simulink model "fcw_ut"  (Simulink 8.1)
settings: Solver=FixedStepDiscrete  StartTime=0.0  StopTime=10.0  FixedStep=5e-3  RelTol=1e-3
undefined symbols (not defined in the file or in its folder): VIFO_BrakePedalPressed_flg, VIFO_FCWTargetVehicleTtcX_ms, VIFO_FCWTargetVehRelSpeedX_mps, VJUD_FCWActionReq_flg, VJUD_FCWDBSAllowed_flg, VJUD_FCWDeactivationReq_flg, VJUD_FCWEnableReq_flg, VJUD_FCWOperational_flg, VJUD_FCWReturnOperational_flg, VJUD_FCWSpeedInRange_flg
libraries: siltestlib x22, hcu_lib x1, fcw x1, simulink x1
settings Model: Creator=xsellart  LastModifiedBy=AT015411
settings DataIOCC: SignalLoggingSaveFormat=Dataset
settings OptimizationCC: ExpressionDepthLimit=128
settings DebuggingCC: FcnCallInpInsideContextMsg=EnableAllAsError
settings GRTTargetCC: CombineOutputUpdateFcns=on  GRTInterface=off

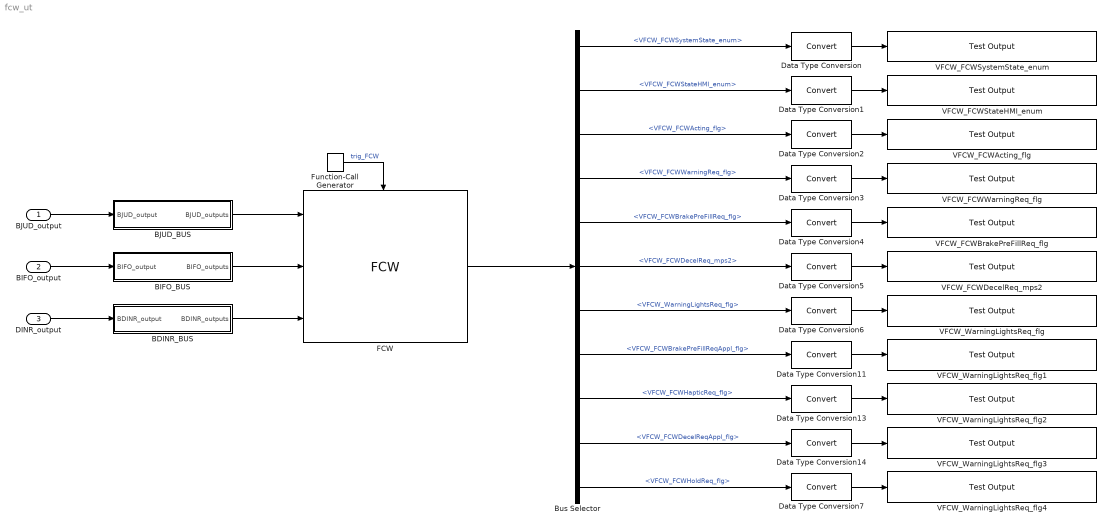
== system fcw_ut ==
  BJUD_output : Inport  OutDataTypeStr=Bus: BJUD_outputs
  BIFO_output : Inport  Port=2  OutDataTypeStr=Bus: BIFO_outputs
  DINR_output : Inport  Port=3  OutDataTypeStr=Bus: BDINR_outputs
  BDINR_BUS : Subsystem
  BIFO_BUS : Subsystem
  BJUD_BUS : Subsystem
  Bus Selector : BusSelector  OutputSignals=VFCW_FCWSystemState_enum,VFCW_FCWStateHMI_enum,VFCW_FCWActing_flg,VFCW_FCWWarningReq_flg,VFCW_FCWBrakePreFillReq_flg,VFCW_FCWDecelReq_mps2,VFCW_WarningLightsReq_flg,VFCW_FCWBrakePreFillReqAppl_flg,VFCW_FCWHapticReq_flg,VFCW_FCWDecelReqAppl_flg,VFCW_FCWHoldReq_flg
  Data Type Conversion{,1..7,11,13..14} (11 alike) : DataTypeConversion
  FCW : fcw/FCW
  Function-Call Generator : simulink/Ports & Subsystems/Function-Call Generator  sample_time=100E-3  numberOfIterations=1
  VFCW_FCWActing_flg : siltestlib/Test Output  varname=VFCW_FCWActing_flg  sampletime=-1
  VFCW_FCWBrakePreFillReq_flg : siltestlib/Test Output  varname=VFCW_FCWBrakePreFillReq_flg  sampletime=-1
  VFCW_FCWDecelReq_mps2 : siltestlib/Test Output  varname=VFCW_FCWDecelReq_mps2  sampletime=-1
  VFCW_FCWStateHMI_enum : siltestlib/Test Output  varname=VFCW_FCWStateHMI_enum  sampletime=-1
  VFCW_FCWSystemState_enum : siltestlib/Test Output  varname=VFCW_FCWSystemState_enum  sampletime=-1
  VFCW_FCWWarningReq_flg : siltestlib/Test Output  varname=VFCW_FCWWarningReq_flg  sampletime=-1
  VFCW_WarningLightsReq_flg : siltestlib/Test Output  varname=VFCW_WarningLightsReq_flg  sampletime=-1
  VFCW_WarningLightsReq_flg1 : siltestlib/Test Output  varname=VFCW_FCWBrakePreFillReqAppl_flg  sampletime=-1
  VFCW_WarningLightsReq_flg2 : siltestlib/Test Output  varname=VFCW_FCWHapticReq_flg  sampletime=-1
  VFCW_WarningLightsReq_flg3 : siltestlib/Test Output  varname=VFCW_FCWDecelReqAppl_flg  sampletime=-1
  VFCW_WarningLightsReq_flg4 : siltestlib/Test Output  varname=VFCW_FCWHoldReq_flg  sampletime=-1
  wires:
  BJUD_output/1 -> BJUD_BUS/1(BJUD_output)
  BIFO_output/1 -> BIFO_BUS/1(BIFO_output)
  DINR_output/1 -> BDINR_BUS/1(BDINR_output)
  FCW/1 -> Bus Selector/1
  BJUD_BUS/1(BJUD_outputs) -> FCW/1
  BIFO_BUS/1(BIFO_outputs) -> FCW/2
  BDINR_BUS/1(BDINR_outputs) -> FCW/3
  Function-Call Generator/1 -> FCW/Trigger  "trig_FCW"
  Bus Selector/1 -> Data Type Conversion/1  "<VFCW_FCWSystemState_enum>"
  Bus Selector/2 -> Data Type Conversion1/1  "<VFCW_FCWStateHMI_enum>"
  Bus Selector/3 -> Data Type Conversion2/1  "<VFCW_FCWActing_flg>"
  Bus Selector/4 -> Data Type Conversion3/1  "<VFCW_FCWWarningReq_flg>"
  Bus Selector/5 -> Data Type Conversion4/1  "<VFCW_FCWBrakePreFillReq_flg>"
  Bus Selector/7 -> Data Type Conversion6/1  "<VFCW_WarningLightsReq_flg>"
  Data Type Conversion/1 -> VFCW_FCWSystemState_enum/1
  Data Type Conversion1/1 -> VFCW_FCWStateHMI_enum/1
  Data Type Conversion2/1 -> VFCW_FCWActing_flg/1
  Data Type Conversion3/1 -> VFCW_FCWWarningReq_flg/1
  Data Type Conversion4/1 -> VFCW_FCWBrakePreFillReq_flg/1
  Data Type Conversion6/1 -> VFCW_WarningLightsReq_flg/1
  Bus Selector/6 -> Data Type Conversion5/1  "<VFCW_FCWDecelReq_mps2>"
  Data Type Conversion5/1 -> VFCW_FCWDecelReq_mps2/1
  Data Type Conversion11/1 -> VFCW_WarningLightsReq_flg1/1
  Bus Selector/8 -> Data Type Conversion11/1  "<VFCW_FCWBrakePreFillReqAppl_flg>"
  Data Type Conversion13/1 -> VFCW_WarningLightsReq_flg2/1
  Bus Selector/9 -> Data Type Conversion13/1  "<VFCW_FCWHapticReq_flg>"
  Data Type Conversion14/1 -> VFCW_WarningLightsReq_flg3/1
  Bus Selector/10 -> Data Type Conversion14/1  "<VFCW_FCWDecelReqAppl_flg>"
  Data Type Conversion7/1 -> VFCW_WarningLightsReq_flg4/1
  Bus Selector/11 -> Data Type Conversion7/1  "<VFCW_FCWHoldReq_flg>"

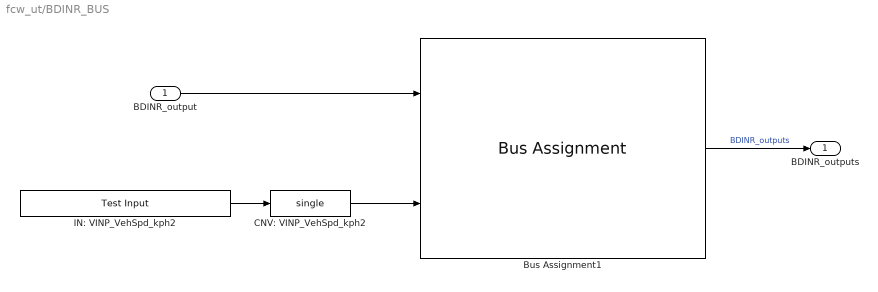
== system fcw_ut/BDINR_BUS ==
  BDINR_output : Inport  OutDataTypeStr=Bus: BDINR_outputs
  Bus Assignment1 : BusAssignment  AssignedSignals=VDINR_VehSpd_mps
  CNV: VINP_VehSpd_kph2 : DataTypeConversion  OutDataTypeStr=single
  IN: VINP_VehSpd_kph2 : siltestlib/Test Input  varname=VDINR_VehSpd_mps  sampletime=-1
  BDINR_outputs : Outport
  wires:
  BDINR_output/1 -> Bus Assignment1/1
  Bus Assignment1/1 -> BDINR_outputs/1  "BDINR_outputs"
  IN: VINP_VehSpd_kph2/1 -> CNV: VINP_VehSpd_kph2/1
  CNV: VINP_VehSpd_kph2/1 -> Bus Assignment1/2

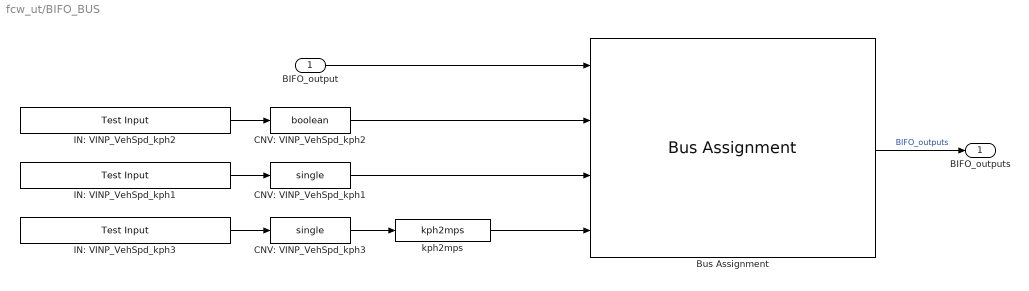
== system fcw_ut/BIFO_BUS ==
  BIFO_output : Inport  OutDataTypeStr=Bus: BIFO_outputs
  Bus Assignment : BusAssignment  AssignedSignals=VIFO_BrakePedalPressed_flg,VIFO_FCWTargetVehicleTtcX_ms,VIFO_FCWTargetVehRelSpeedX_mps
  CNV: VINP_VehSpd_kph1 : DataTypeConversion  OutDataTypeStr=single
  CNV: VINP_VehSpd_kph2 : DataTypeConversion  OutDataTypeStr=boolean
  CNV: VINP_VehSpd_kph3 : DataTypeConversion  OutDataTypeStr=single
  IN: VINP_VehSpd_kph1 : siltestlib/Test Input  varname=VIFO_FCWTargetVehicleTtcX_ms  sampletime=-1
  IN: VINP_VehSpd_kph2 : siltestlib/Test Input  varname=VIFO_BrakePedalPressed_flg  sampletime=-1
  IN: VINP_VehSpd_kph3 : siltestlib/Test Input  varname=VIFO_FCWTargetVehRelSpeed_kph  sampletime=-1
  kph2mps : hcu_lib/kph2mps
  BIFO_outputs : Outport
  wires:
  CNV: VINP_VehSpd_kph1/1 -> Bus Assignment/3
  CNV: VINP_VehSpd_kph3/1 -> kph2mps/1
  IN: VINP_VehSpd_kph3/1 -> CNV: VINP_VehSpd_kph3/1
  IN: VINP_VehSpd_kph1/1 -> CNV: VINP_VehSpd_kph1/1
  CNV: VINP_VehSpd_kph2/1 -> Bus Assignment/2
  IN: VINP_VehSpd_kph2/1 -> CNV: VINP_VehSpd_kph2/1
  Bus Assignment/1 -> BIFO_outputs/1  "BIFO_outputs"
  BIFO_output/1 -> Bus Assignment/1
  kph2mps/1 -> Bus Assignment/4

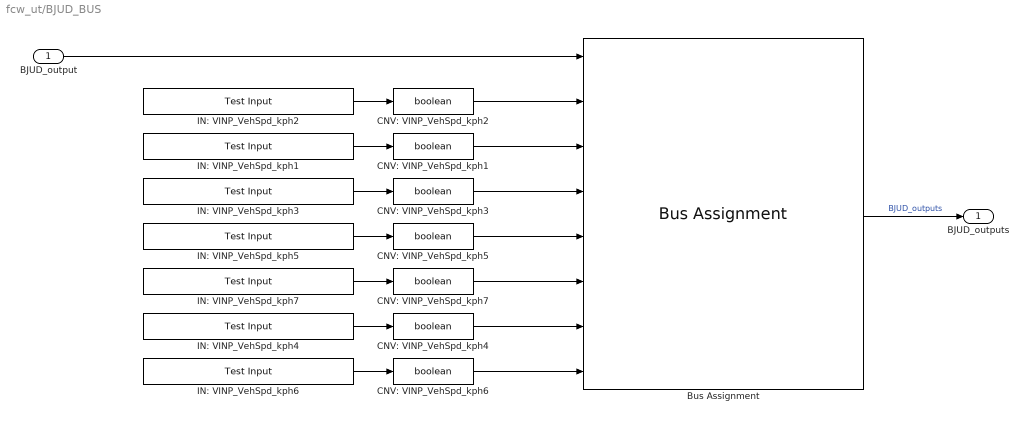
== system fcw_ut/BJUD_BUS ==
  BJUD_output : Inport  OutDataTypeStr=Bus: BJUD_outputs
  Bus Assignment : BusAssignment  AssignedSignals=VJUD_FCWEnableReq_flg,VJUD_FCWOperational_flg,VJUD_FCWSpeedInRange_flg,VJUD_FCWActionReq_flg,VJUD_FCWReturnOperational_flg,VJUD_FCWDeactivationReq_flg,VJUD_FCWDBSAllowed_flg
  CNV: VINP_VehSpd_kph{1..7} (7 alike) : DataTypeConversion  OutDataTypeStr=boolean
  IN: VINP_VehSpd_kph1 : siltestlib/Test Input  varname=VJUD_FCWOperational_flg  sampletime=-1
  IN: VINP_VehSpd_kph2 : siltestlib/Test Input  varname=VJUD_FCWEnableReq_flg  sampletime=-1
  IN: VINP_VehSpd_kph3 : siltestlib/Test Input  varname=VJUD_FCWSpeedInRange_flg  sampletime=-1
  IN: VINP_VehSpd_kph4 : siltestlib/Test Input  varname=VJUD_FCWDeactivationReq_flg  sampletime=-1
  IN: VINP_VehSpd_kph5 : siltestlib/Test Input  varname=VJUD_FCWActionReq_flg  sampletime=-1
  IN: VINP_VehSpd_kph6 : siltestlib/Test Input  varname=VJUD_FCWDBSAllowed_flg  sampletime=-1
  IN: VINP_VehSpd_kph7 : siltestlib/Test Input  varname=VJUD_FCWReturnOperational_flg  sampletime=-1
  BJUD_outputs : Outport
  wires:
  BJUD_output/1 -> Bus Assignment/1
  Bus Assignment/1 -> BJUD_outputs/1  "BJUD_outputs"
  IN: VINP_VehSpd_kph2/1 -> CNV: VINP_VehSpd_kph2/1
  CNV: VINP_VehSpd_kph2/1 -> Bus Assignment/2
  IN: VINP_VehSpd_kph1/1 -> CNV: VINP_VehSpd_kph1/1
  IN: VINP_VehSpd_kph3/1 -> CNV: VINP_VehSpd_kph3/1
  CNV: VINP_VehSpd_kph3/1 -> Bus Assignment/4
  CNV: VINP_VehSpd_kph1/1 -> Bus Assignment/3
  IN: VINP_VehSpd_kph5/1 -> CNV: VINP_VehSpd_kph5/1
  IN: VINP_VehSpd_kph4/1 -> CNV: VINP_VehSpd_kph4/1
  IN: VINP_VehSpd_kph6/1 -> CNV: VINP_VehSpd_kph6/1
  CNV: VINP_VehSpd_kph5/1 -> Bus Assignment/5
  CNV: VINP_VehSpd_kph7/1 -> Bus Assignment/6
  CNV: VINP_VehSpd_kph4/1 -> Bus Assignment/7
  CNV: VINP_VehSpd_kph6/1 -> Bus Assignment/8
  IN: VINP_VehSpd_kph7/1 -> CNV: VINP_VehSpd_kph7/1
